simulink model "longtitudinalmodel"  (R2022b)
settings: Solver=VariableStepAuto  StartTime=0.0  StopTime=10.0  FixedStep=0.01  RelTol=1e-3
InitFcn:
  | vehicle_longitudinal_para
values from neighbouring files (symbols this model uses):
  engine_cmd = [0.1, 0.2, 0.3, 0.4, 0.5, 0.4, 0.4, 0.5, 0.4, 0.3]    [vehicle_longitudinal_para.m]
  FR = 1.18    [VehicleLongtitudinalModel.m]    (also in vehicle_longitudinal_para.m)
  generator_cmd = [0, 1, 2, 3, 4, 5, 6, 7, 8, 9] * 5    [vehicle_longitudinal_para.m]
  k = Nr/Ns    (= 2.6)    [VehicleLongtitudinalModel.m]    (also in vehicle_longitudinal_para.m)
  motor_cmd = 1000 + 20 * [0, 1, 2, 3, 4, 5, 6, 7, 8, 9]    [vehicle_longitudinal_para.m]
  R_tire = 0.5    [VehicleLongtitudinalModel.m]    (also in vehicle_longitudinal_para.m)
  testTime = [0, 1, 2, 3, 4, 5, 6, 7, 8, 9]    [vehicle_longitudinal_para.m]
settings Model: Creator=12159  LastModifiedBy=12159

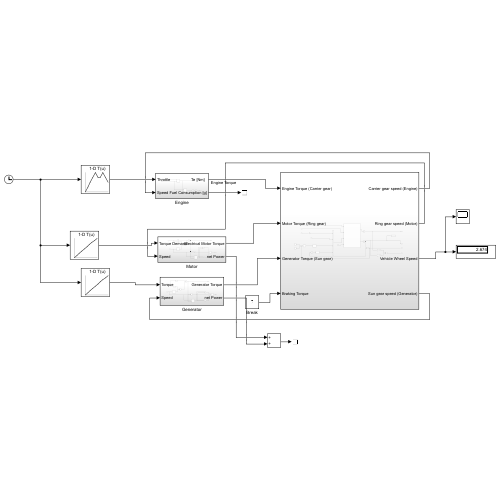
[thumbnail: Simulink's stored preview of the top-level diagram]
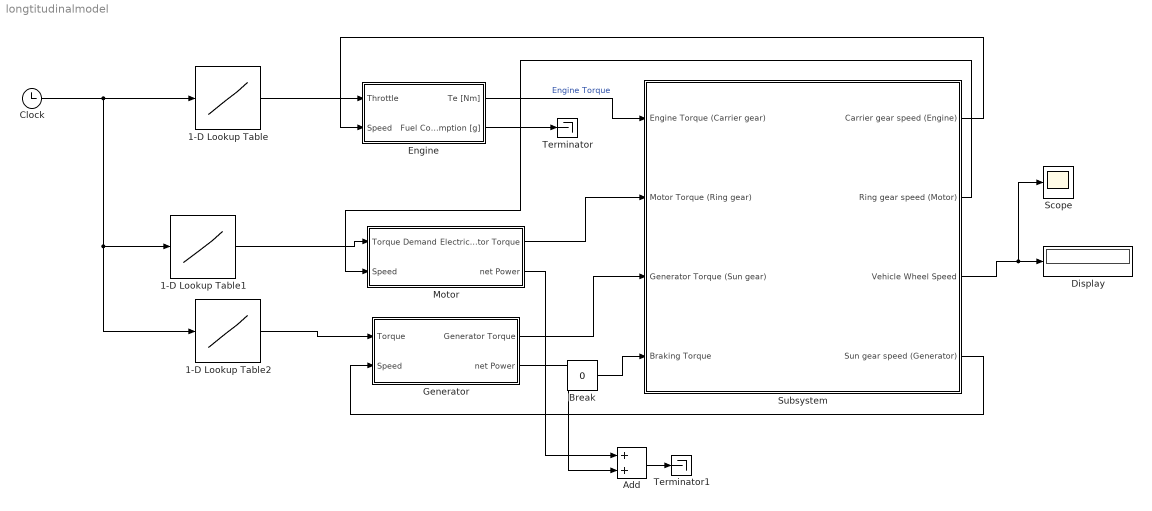
== system longtitudinalmodel ==
  1-D Lookup Table : Lookup_n-D  NumberOfTableDimensions=1  BreakpointsForDimension1=testTime  Table=engine_cmd  InternalRulePriority=Speed  RndMeth=Simplest
  1-D Lookup Table1 : Lookup_n-D  NumberOfTableDimensions=1  BreakpointsForDimension1=testTime  Table=motor_cmd  InternalRulePriority=Speed  RndMeth=Simplest
  1-D Lookup Table2 : Lookup_n-D  NumberOfTableDimensions=1  BreakpointsForDimension1=testTime  Table=generator_cmd  InternalRulePriority=Speed  RndMeth=Simplest
  Add : Sum
  Break : Constant  Value=0
  Clock : Clock
  Display : Display
  Engine : Subsystem
  Generator : Subsystem
  Motor : Subsystem
  Scope : Scope
  Subsystem : Subsystem
  Terminator : Terminator
  Terminator1 : Terminator
  wires:
  Clock/1 -> 1-D Lookup Table/1, 1-D Lookup Table1/1, 1-D Lookup Table2/1
  1-D Lookup Table/1 -> Engine/1(Throttle)
  1-D Lookup Table1/1 -> Motor/1(Torque Demand)
  Motor/2(net Power) -> Add/1
  Generator/2(net Power) -> Add/2
  Add/1 -> Terminator1/1
  1-D Lookup Table2/1 -> Generator/1(Torque)
  Engine/2(Fuel Consumption [g]) -> Terminator/1
  Engine/1("Te [Nm] ") -> Subsystem/1(Engine Torque (Carrier gear))  "Engine Torque"
  Subsystem/1(Carrier gear speed (Engine)) -> Engine/2(Speed)
  Motor/1(Electrical Motor Torque) -> Subsystem/2(Motor Torque (Ring gear))
  Generator/1(Generator Torque) -> Subsystem/3(Generator Torque (Sun gear))
  Break/1 -> Subsystem/4(Braking Torque)
  Subsystem/4(Sun gear speed (Generator)) -> Generator/2(Speed)
  Subsystem/3(Vehicle Wheel Speed) -> Scope/1, Display/1
  Subsystem/2(Ring gear speed (Motor)) -> Motor/2(Speed)

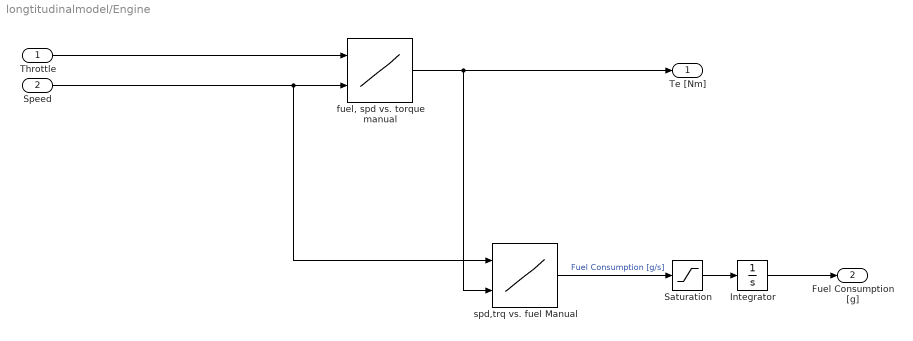
== system longtitudinalmodel/Engine ==
  Throttle : Inport
  Speed : Inport  Port=2
  Integrator : Integrator
  Saturation : Saturate  UpperLimit=1  LowerLimit=0
  "fuel, spd vs. torque manual" : Lookup_n-D  BreakpointsForDimension1=[0 0.1 0.2 0.3 0.4 0.5 0.6 0.7 0.8 0.9 1]  BreakpointsForDimension2=[52.35 55 57.6 60.2 62.85 65.45 68.05 70.7 73.3 75.9 78.55 81.15 83.8 86.4 89 91.65 94.25 96.85 99.5 102.1 104.7 107.35 109.95 112.55 115.2 117.8 120.45 123.05 125.65 128.3 130.9 133.5 136.15 138.75 141.35 144 146.6 149.25 151.85 154.45 157.1 159.7 162.3 164.95 167.55 170.15 172.8 175.4 178 180.65 183.25 185.9 188.5 191.1 193.75 196.35 198.95 201.6 204.2 206.8 209.45]  Table=[0 0 0 0 0 0 0 0 0 0 0 0 0 0 0 0 0 0 0 0 0 0 0 0 0 0 0 0 0 0 0 0 0 0 0 0 0 0 0 0 0 0 0 0 0 0 0 0 0 0 0 0 0 0 0 0 0 0 0 0 0;106.452310717797 107.649950835792 108.847590953786 110.04523107178 111.242871189774 112.440511307768 113.362831858407 114.051130776794 114.739429695182 115.427728613569 116.116027531957 116.776794493609 117.286135693215 117.80924287119 118.318584070796 118.827925270403 119.351032448378 119.942969518191 120.589970501475 121.250737463127 121.897738446411 122.544739429695 123.164208456244 123.604719764012 124.04523107178 124.485742379548 124.940019665683 125.380530973451 125.821042281219 126.275319567355 126.715830875123 127.170108161259 127.610619469027 128.064896755162 128.50540806293 128.945919370698 129.386430678466 129.840707964602 130.28121927237 130.721730580138 131.176007866273 131.616519174041 132.057030481809 132.511307767945 132.951819075713 133.392330383481 133.832841691249 134.287118977384 134.727630285152 135.16814159292 135.622418879056 136.062930186824 136.51720747296 136.957718780728 137.398230088496 137.935103244838 138.34808259587 138.89872173058 139.44936086529 140 140.412979351032;212.904621435595 215.299901671583 217.695181907571 220.09046214356 222.485742379548 224.881022615536 226.725663716814 228.102261553589 229.478859390364 230.855457227139 232.232055063913 233.553588987217 234.572271386431 235.61848574238 236.637168141593 237.655850540806 238.702064896755 239.885939036382 241.17994100295 242.501474926254 243.795476892822 245.08947885939 246.328416912488 247.209439528024 248.09046214356 248.971484759095 249.880039331367 250.761061946903 251.642084562439 252.55063913471 253.431661750246 254.340216322517 255.221238938053 256.129793510324 257.01081612586 257.891838741396 258.772861356932 259.681415929204 260.562438544739 261.443461160275 262.352015732547 263.233038348083 264.114060963618 265.02261553589 265.903638151426 266.784660766962 267.665683382498 268.574237954769 269.455260570305 270.336283185841 271.244837758112 272.125860373648 273.034414945919 273.915437561455 274.796460176991 275.870206489676 276.69616519174 277.79744346116 278.89872173058 280 280.825958702065;319.356932153392 322.949852507375 326.542772861357 330.135693215339 333.728613569322 337.321533923304 340.088495575221 342.153392330383 344.218289085546 346.283185840708 348.34808259587 350.330383480826 351.858407079646 353.427728613569 354.955752212389 356.483775811209 358.053097345133 359.828908554572 361.769911504425 363.75221238938 365.693215339233 367.634218289085 369.492625368732 370.814159292035 372.135693215339 373.457227138643 374.82005899705 376.141592920354 377.463126843658 378.825958702065 380.147492625369 381.510324483776 382.83185840708 384.194690265487 385.516224188791 386.837758112094 388.159292035398 389.522123893805 390.843657817109 392.165191740413 393.52802359882 394.849557522124 396.171091445428 397.533923303835 398.855457227139 400.176991150442 401.498525073746 402.861356932153 404.182890855457 405.504424778761 406.867256637168 408.188790560472 409.551622418879 410.873156342183 412.194690265487 413.805309734513 415.044247787611 416.69616519174 418.34808259587 420 421.238938053097;425.80924287119 430.599803343166 435.390363815143 440.180924287119 444.971484759095 449.762045231072 453.451327433628 456.204523107178 458.957718780728 461.710914454277 464.464110127827 467.107177974435 469.144542772861 471.236971484759 473.274336283186 475.311701081613 477.40412979351 479.771878072763 482.3598820059 485.002949852507 487.590953785644 490.178957718781 492.656833824975 494.418879056047 496.180924287119 497.942969518191 499.760078662734 501.522123893805 503.284169124877 505.10127826942 506.863323500492 508.680432645034 510.442477876106 512.259587020649 514.021632251721 515.783677482793 517.545722713864 519.362831858407 521.124877089479 522.886922320551 524.704031465093 526.466076696165 528.228121927237 530.04523107178 531.807276302852 533.569321533923 535.331366764995 537.148475909538 538.91052114061 ...(+6299 chars)]  InternalRulePriority=Speed  RndMeth=Simplest
      settings: InputPortMap=u0,u1
  spd,trq vs. fuel Manual : Lookup_n-D  BreakpointsForDimension1=[52.35 55 57.6 60.2 62.85 65.45 68.05 70.7 73.3 75.9 78.55 81.15 83.8 86.4 89 91.65 94.25 96.85 99.5 102.1 104.7 107.35 109.95 112.55 115.2 117.8 120.45 123.05 125.65 128.3 130.9 133.5 136.15 138.75 141.35 144 146.6 149.25 151.85 154.45 157.1 159.7 162.3 164.95 167.55 170.15 172.8 175.4 178 180.65 183.25 185.9 188.5 191.1 193.75 196.35 198.95 201.6 204.2 206.8 209.45]  BreakpointsForDimension2=[0 137.659783677483 206.489675516224 275.319567354966 344.149459193707 412.979351032448 481.80924287119 550.639134709931 619.469026548673 688.298918387414 757.128810226155 825.958702064897 894.788593903638 963.618485742379 1032.44837758112 1101.27826941986 1170.1081612586 1238.93805309735 1307.76794493609 1376.59783677483]  Table=[0 3.924 1.968 1.428 1.392 1.542 1.74 1.938 2.118 2.286 2.442 2.61 2.79 3.006 3.27 3.594 3.99 4.476 5.052 5.742;0 4.002 2.052 1.518 1.494 1.65 1.854 2.058 2.25 2.424 2.592 2.76 2.952 3.18 3.45 3.78 4.182 4.674 5.262 5.958;0 4.074 2.13 1.608 1.59 1.752 1.962 2.178 2.376 2.556 2.73 2.91 3.108 3.342 3.618 3.954 4.368 4.866 5.46 6.18;0 4.146 2.208 1.692 1.68 1.848 2.07 2.292 2.496 2.682 2.862 3.054 3.258 3.498 3.78 4.128 4.548 5.052 5.652 6.36;0 4.206 2.28 1.77 1.764 1.944 2.172 2.4 2.61 2.808 2.994 3.186 3.402 3.648 3.942 4.296 4.722 5.232 5.844 6.54;0 4.266 2.346 1.842 1.848 2.052 2.28 2.508 2.706 2.898 3.09 3.324 3.54 3.792 4.092 4.452 4.89 5.406 6 6.72;0 4.326 2.412 1.92 1.926 2.154 2.382 2.616 2.844 3.036 3.228 3.48 3.732 3.936 4.242 4.614 5.052 5.58 6.18 6.96;0 4.386 2.478 1.986 2.004 2.226 2.478 2.718 2.952 3.168 3.354 3.588 3.894 4.08 4.392 4.764 5.214 5.748 6.36 7.14;0 4.44 2.538 2.058 2.082 2.298 2.55 2.796 3.048 3.288 3.474 3.702 4.008 4.302 4.536 4.92 5.37 5.91 6.54 7.32;0 4.494 2.598 2.124 2.154 2.37 2.622 2.868 3.12 3.366 3.582 3.816 4.122 4.428 4.68 5.064 5.526 6.06 6.72 7.5;0 4.548 2.658 2.196 2.232 2.442 2.688 2.94 3.192 3.462 3.666 3.936 4.248 4.56 4.818 5.214 5.682 6.24 6.9 7.62;0 4.602 2.718 2.262 2.304 2.514 2.76 3.012 3.276 3.564 3.768 4.056 4.368 4.686 4.992 5.358 5.832 6.42 7.08 7.8;0 4.656 2.784 2.328 2.376 2.58 2.832 3.096 3.378 3.666 3.888 4.182 4.482 4.8 5.112 5.502 5.982 6.54 7.2 7.98;0 4.71 2.844 2.394 2.454 2.652 2.91 3.198 3.486 3.768 4.014 4.308 4.602 4.914 5.22 5.646 6.12 6.72 7.38 8.16;0 4.77 2.904 2.466 2.526 2.73 3.018 3.3 3.588 3.87 4.14 4.428 4.722 5.028 5.34 5.82 6.3 6.84 7.56 8.34;0 4.824 2.97 2.532 2.544 2.832 3.12 3.402 3.69 3.978 4.272 4.578 4.878 5.184 5.508 5.892 6.42 7.02 7.68 8.46;0 4.884 3.036 2.604 2.676 2.952 3.24 3.528 3.81 4.104 4.428 4.758 5.082 5.406 5.712 6.12 6.6 7.14 7.86 8.64;0 4.944 3.102 2.676 2.778 3.078 3.36 3.648 3.93 4.23 4.554 4.878 5.208 5.532 5.868 6.3 6.84 7.32 8.04 8.82;0 5.004 3.168 2.748 2.808 3.174 3.432 3.768 4.056 4.35 4.68 5.004 5.328 5.67 6 6.42 6.96 7.5 8.16 9;0 5.07 3.24 2.826 2.916 3.192 3.624 3.768 4.176 4.476 4.8 5.13 5.466 5.814 6.18 6.54 7.08 7.62 8.34 9.12;0 5.136 3.312 2.904 3 3.3 3.63 3.954 4.296 4.602 4.926 5.268 5.616 5.964 6.3 6.66 7.2 7.8 8.52 9.3;0 5.208 3.384 2.982 3.084 3.384 3.72 4.05 4.374 4.722 5.07 5.418 5.766 6.12 6.48 6.78 7.32 7.92 8.64 9.48;0 5.28 3.462 3.066 3.174 3.462 3.822 4.134 4.488 4.86 5.214 5.562 5.91 6.24 6.6 6.96 7.5 8.1 8.82 9.66;0 5.352 3.54 3.15 3.264 3.552 3.912 4.248 4.596 5.064 5.34 5.694 6.06 6.42 6.78 7.08 7.62 8.28 9 9.84;0 5.43 3.618 3.234 3.354 3.654 4.002 4.344 4.716 5.304 5.544 5.814 6.18 6.54 6.9 7.26 7.74 8.4 9.12 9.96;0 5.508 3.708 3.324 3.45 3.75 4.104 4.476 4.824 5.562 5.76 6 6.3 6.66 7.02 7.38 7.86 8.58 9.3 10.14;0 5.592 3.792 3.414 3.546 3.852 4.212 4.59 4.95 5.34 5.958 6.24 6.48 6.78 7.14 7.56 8.1 8.7 9.48 10.32;0 5.676 3.882 3.51 3.642 3.96 4.32 4.71 5.058 5.454 6.18 6.48 6.72 6.9 7.26 7.8 8.34 8.82 9.66 10.5;0 5.766 3.978 3.612 3.75 4.068 4.434 4.824 5.166 5.574 6.42 6.66 6.96 7.14 7.44 7.98 8.52 9 9.78 10.68;0 5.856 4.074 3.714 3.852 4.176 4.548 4.92 5.292 5.706 6.66 6.84 7.14 7.38 7.62 8.1 8.64 9.18 9.96 10.86;0 5.952 4.176 3.816 3.96 4.29 4.668 5.046 5.418 5.826 6.264 6.702 7.38 7.62 7.86 8.22 8.76 9.36 10.14 10.98;0 6.06 4.278 3.924 4.074 4.404 4.788 5.166 5.538 5.94 6.39 6.834 7.56 7.86 8.1 8.4 8.88 9.54 10.32 11.16;0 6.18 4.386 4.038 4.188 4.524 4.908 5.298 5.67 6.06 6.516 6.972 7.74 8.04 8.34 8.58 9.06 9.72 10.5 11.34;0 6.24 4.494 4.152 4.308 4.65 5.04 5.43 5.802 6.18 6.642 7.134 7.98 8.28 8.52 8.82 9.18 9.9 10.68 11.52;0 6.36 4.608 4.266 4.428 4.776 5.166 5.562 5.94 6.3 6.762 7.266 8.16 8.46 8.76 9 9.36 10.08 10.86 11.7;0 6.48 4.728 4.392 4.554 4.902 5.298 5.7 6.06 6.42 6.888 7.398 8.4 8.64 8.94 9.24 9.48 10.32 11.04 11.88;0 6.6 4.848 4.518 4.686 5.034 5.436 5.838 6.24 6.6 7.014 7.506 8.004 8.586 9.126 9.42 9.72 10.5 11.22 12.06;0 6.72 4.974 4.644 4.818 5.172 5.58 5.982 6.36 6.72 7.14 ...(+2461 chars)]  InternalRulePriority=Speed  RndMeth=Simplest
      settings: InputPortMap=u0,u1
  "Te [Nm] " : Outport
  Fuel Consumption [g] : Outport  Port=2
  wires:
  Integrator/1 -> Fuel Consumption [g]/1
  "fuel, spd vs. torque manual"/1 -> "Te [Nm] "/1, spd,trq vs. fuel Manual/2
  Throttle/1 -> "fuel, spd vs. torque manual"/1
  Speed/1 -> spd,trq vs. fuel Manual/1, "fuel, spd vs. torque manual"/2
  spd,trq vs. fuel Manual/1 -> Saturation/1  "Fuel Consumption [g/s]"
  Saturation/1 -> Integrator/1

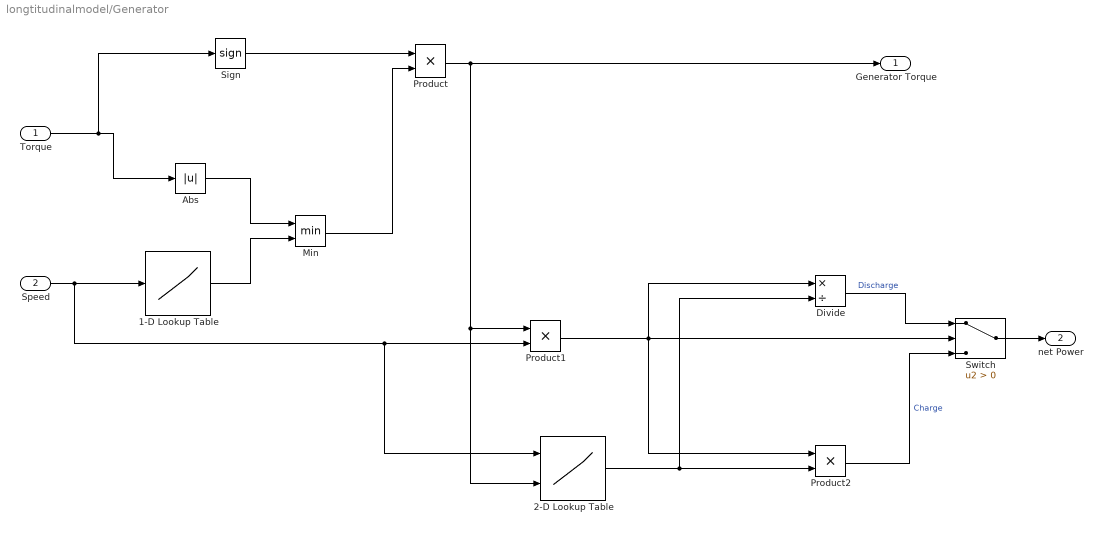
== system longtitudinalmodel/Generator ==
  Torque : Inport
  Speed : Inport  Port=2
  1-D Lookup Table : Lookup_n-D  NumberOfTableDimensions=1  BreakpointsForDimension1=[-20943.951023932 -1047.1975511966 -837.758040957278 -680.678408277789 -575.958653158129 -418.879020478639 -366.519142918809 -314.159265358979 -261.799387799149 -209.43951023932 -157.07963267949 -104.71975511966 -52.3598775598299 0 52.3598775598299 104.71975511966 157.07963267949 209.43951023932 261.799387799149 314.159265358979 366.519142918809 418.879020478639 575.958653158129 680.678408277789 837.758040957278 1047.1975511966 20943.951023932]  Table=[0.012 17.16 21.6 26.4 31.2 43.2 49.2 57.6 66 66 66 66 66 66 66 66 66 66 66 57.6 49.2 43.2 31.2 26.4 21.6 17.16 0.012]  InternalRulePriority=Speed  RndMeth=Simplest
  2-D Lookup Table : Lookup_n-D  BreakpointsForDimension1=[-628.318530717959 -575.958653158129 -418.879020478639 -366.519142918809 -314.159265358979 -261.799387799149 -209.43951023932 -157.07963267949 -104.71975511966 -52.3598775598299 0 52.3598775598299 104.71975511966 157.07963267949 209.43951023932 261.799387799149 314.159265358979 366.519142918809 418.879020478639 575.958653158129 628.318530717959]  BreakpointsForDimension2=[-55 -45 -35 -25 -15 -5 0 5 15 25 35 45 55]  Table=[0.836 0.8455 0.855 0.8645 0.855 0.7505 0.7505 0.7505 0.855 0.8645 0.855 0.8455 0.836;0.836 0.8455 0.855 0.8645 0.855 0.7505 0.7505 0.7505 0.855 0.8645 0.855 0.8455 0.836;0.836 0.8455 0.855 0.8645 0.855 0.7505 0.7505 0.7505 0.855 0.8645 0.855 0.8455 0.836;0.8265 0.836 0.855 0.855 0.855 0.76 0.76 0.76 0.855 0.855 0.855 0.836 0.8265;0.8075 0.8265 0.8455 0.855 0.855 0.7695 0.7695 0.7695 0.855 0.855 0.8455 0.8265 0.8075;0.7885 0.8075 0.8265 0.8455 0.8455 0.779 0.779 0.779 0.8455 0.8455 0.8265 0.8075 0.7885;0.76 0.7885 0.8075 0.8265 0.8455 0.779 0.779 0.779 0.8455 0.8265 0.8075 0.7885 0.76;0.722 0.7505 0.779 0.8075 0.8265 0.779 0.779 0.779 0.8265 0.8075 0.779 0.7505 0.722;0.646 0.684 0.722 0.76 0.798 0.7695 0.76 0.7695 0.798 0.76 0.722 0.684 0.646;0.494 0.5415 0.5985 0.6555 0.7315 0.76 0.76 0.76 0.7315 0.6555 0.5985 0.5415 0.494;0.494 0.5415 0.5985 0.6555 0.7315 0.76 0.76 0.76 0.7315 0.6555 0.5985 0.5415 0.494;0.494 0.5415 0.5985 0.6555 0.7315 0.76 0.76 0.76 0.7315 0.6555 0.5985 0.5415 0.494;0.646 0.684 0.722 0.76 0.798 0.7695 0.76 0.7695 0.798 0.76 0.722 0.684 0.646;0.722 0.7505 0.779 0.8075 0.8265 0.779 0.779 0.779 0.8265 0.8075 0.779 0.7505 0.722;0.76 0.7885 0.8075 0.8265 0.8455 0.779 0.779 0.779 0.8455 0.8265 0.8075 0.7885 0.76;0.7885 0.8075 0.8265 0.8455 0.8455 0.779 0.779 0.779 0.8455 0.8455 0.8265 0.8075 0.7885;0.8075 0.8265 0.8455 0.855 0.855 0.7695 0.7695 0.7695 0.855 0.855 0.8455 0.8265 0.8075;0.8265 0.836 0.855 0.855 0.855 0.76 0.76 0.76 0.855 0.855 0.855 0.836 0.8265;0.836 0.8455 0.855 0.8645 0.855 0.7505 0.7505 0.7505 0.855 0.8645 0.855 0.8455 0.836;0.836 0.8455 0.855 0.8645 0.855 0.7505 0.7505 0.7505 0.855 0.8645 0.855 0.8455 0.836;0.836 0.8455 0.855 0.8645 0.855 0.7505 0.7505 0.7505 0.855 0.8645 0.855 0.8455 0.836]  InternalRulePriority=Speed  RndMeth=Simplest
      settings: InputPortMap=u0,u1
  Abs : Abs  SaturateOnIntegerOverflow=off
  Divide : Product  Inputs=*/
  Min : MinMax  Inputs=2
  Product : Product
  Product1 : Product
  Product2 : Product
  Sign : Signum
  Switch : Switch  Criteria=u2 > Threshold  SaturateOnIntegerOverflow=off  InputSameDT=off
  Generator Torque : Outport
  net Power : Outport  Port=2
  wires:
  Speed/1 -> 2-D Lookup Table/1, Product1/2, 1-D Lookup Table/1
  1-D Lookup Table/1 -> Min/2
  Torque/1 -> Sign/1, Abs/1
  Sign/1 -> Product/1
  Min/1 -> Product/2
  Abs/1 -> Min/1
  Product/1 -> 2-D Lookup Table/2, Product1/1, Generator Torque/1
  2-D Lookup Table/1 -> Divide/2, Product2/2
  Product1/1 -> Product2/1, Divide/1, Switch/2
  Product2/1 -> Switch/3  "Charge"
  Divide/1 -> Switch/1  "Discharge"
  Switch/1 -> net Power/1

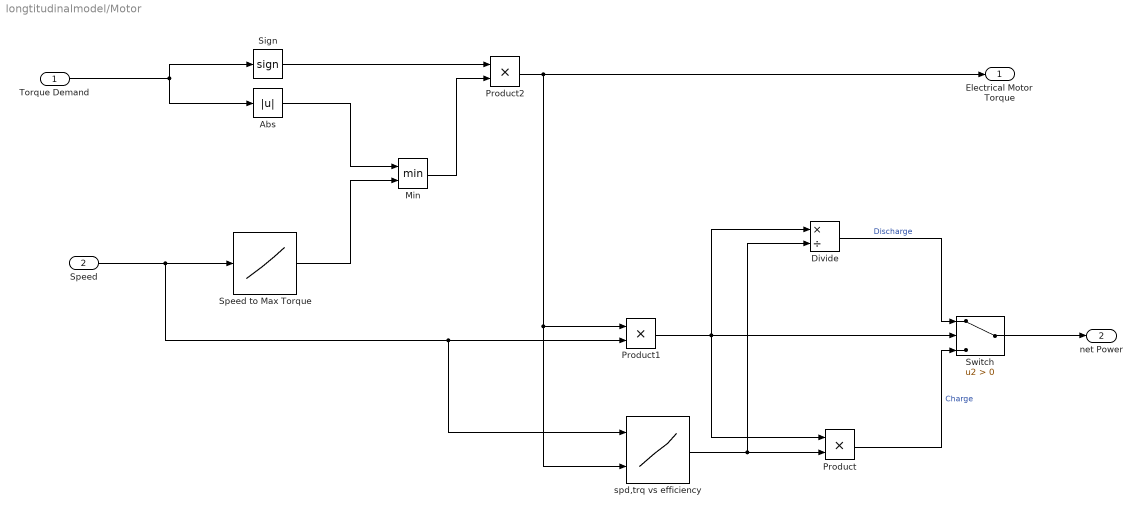
== system longtitudinalmodel/Motor ==
  Torque Demand : Inport
  Speed : Inport  Port=2
  Abs : Abs  SaturateOnIntegerOverflow=off
  Divide : Product  Inputs=*/
  Min : MinMax  Inputs=2
  Product : Product
  Product1 : Product
  Product2 : Product
  Sign : Signum
  Speed to Max Torque : Lookup_n-D  NumberOfTableDimensions=1  BreakpointsForDimension1=[0 52.3598775598299 104.71975511966 157.07963267949 209.43951023932 261.799387799149 314.159265358979 366.519142918809 418.879020478639 471.238898038469 628.318530717959]  Table=[2033.33333333333 2033.33333333333 1929.50354609929 1281.29078014184 959.13475177305 766.099290780142 637.659574468085 546.113475177305 478.099290780142 431.559322033898 318]  InternalRulePriority=Speed  RndMeth=Simplest
  Switch : Switch  Criteria=u2 > Threshold  SaturateOnIntegerOverflow=off  InputSameDT=off
  spd,trq vs efficiency : Lookup_n-D  BreakpointsForDimension1=[0 52.3598775598299 104.71975511966 157.07963267949 209.43951023932 261.799387799149 314.159265358979 366.519142918809 418.879020478639 471.238898038469 628.318530717959]  BreakpointsForDimension2=[-2033.33333333333 -1833.33333333333 -1633.33333333333 -1433.33333333333 -1233.33333333333 -1033.33333333333 -833.333333333333 -633.333333333333 -433.333333333333 -233.333333333333 -33.3333333333333 0 33.3333333333333 233.333333333333 433.333333333333 633.333333333333 833.333333333333 1033.33333333333 1233.33333333333 1433.33333333333 1633.33333333333 1833.33333333333 2033.33333333333]  Table=[0.85975 0.85975 0.85975 0.85975 0.85975 0.85975 0.85975 0.85975 0.85975 0.85975 0.85975 0.85975 0.85975 0.85975 0.85975 0.85975 0.85975 0.85975 0.85975 0.85975 0.85975 0.85975 0.85975;0.532 0.5605 0.589 0.6175 0.646 0.684 0.722 0.76 0.8075 0.855 0.8265 0.85975 0.8265 0.855 0.8075 0.76 0.722 0.684 0.646 0.6175 0.589 0.5605 0.532;0.684 0.703 0.722 0.741 0.7695 0.7885 0.817 0.8455 0.8645 0.893 0.8075 0.85975 0.8075 0.893 0.8645 0.8455 0.817 0.7885 0.7695 0.741 0.722 0.703 0.684;0.684 0.703 0.722 0.741 0.817 0.836 0.855 0.874 0.8835 0.893 0.7885 0.85975 0.7885 0.893 0.8835 0.874 0.855 0.836 0.817 0.741 0.722 0.703 0.684;0.684 0.703 0.722 0.741 0.817 0.836 0.874 0.8835 0.9025 0.9025 0.779 0.85975 0.779 0.9025 0.9025 0.8835 0.874 0.836 0.817 0.741 0.722 0.703 0.684;0.684 0.703 0.722 0.741 0.817 0.836 0.874 0.893 0.9025 0.9025 0.7695 0.85975 0.7695 0.9025 0.9025 0.893 0.874 0.836 0.817 0.741 0.722 0.703 0.684;0.684 0.703 0.722 0.741 0.817 0.836 0.874 0.9025 0.912 0.9025 0.7695 0.85975 0.7695 0.9025 0.912 0.9025 0.874 0.836 0.817 0.741 0.722 0.703 0.684;0.684 0.703 0.722 0.741 0.817 0.836 0.874 0.9025 0.912 0.9025 0.76 0.85975 0.76 0.9025 0.912 0.9025 0.874 0.836 0.817 0.741 0.722 0.703 0.684;0.684 0.703 0.722 0.741 0.817 0.836 0.874 0.9025 0.9025 0.9025 0.76 0.85975 0.76 0.9025 0.9025 0.9025 0.874 0.836 0.817 0.741 0.722 0.703 0.684;0.684 0.703 0.722 0.741 0.817 0.836 0.874 0.9025 0.9025 0.9025 0.7505 0.85975 0.7505 0.9025 0.9025 0.9025 0.874 0.836 0.817 0.741 0.722 0.703 0.684;0.684 0.703 0.722 0.741 0.817 0.836 0.874 0.9025 0.9025 0.9025 0.7505 0.85975 0.7505 0.9025 0.9025 0.9025 0.874 0.836 0.817 0.741 0.722 0.703 0.684]  InternalRulePriority=Speed  RndMeth=Simplest
      settings: InputPortMap=u0,u1
  Electrical Motor Torque : Outport
  net Power : Outport  Port=2
  wires:
  Speed to Max Torque/1 -> Min/2
  Abs/1 -> Min/1
  Torque Demand/1 -> Sign/1, Abs/1
  Sign/1 -> Product2/1
  Min/1 -> Product2/2
  Product2/1 -> Product1/1, spd,trq vs efficiency/2, Electrical Motor Torque/1
  spd,trq vs efficiency/1 -> Divide/2, Product/2
  Switch/1 -> net Power/1
  Speed/1 -> spd,trq vs efficiency/1, Product1/2, Speed to Max Torque/1
  Product1/1 -> Divide/1, Product/1, Switch/2
  Divide/1 -> Switch/1  "Discharge"
  Product/1 -> Switch/3  "Charge"

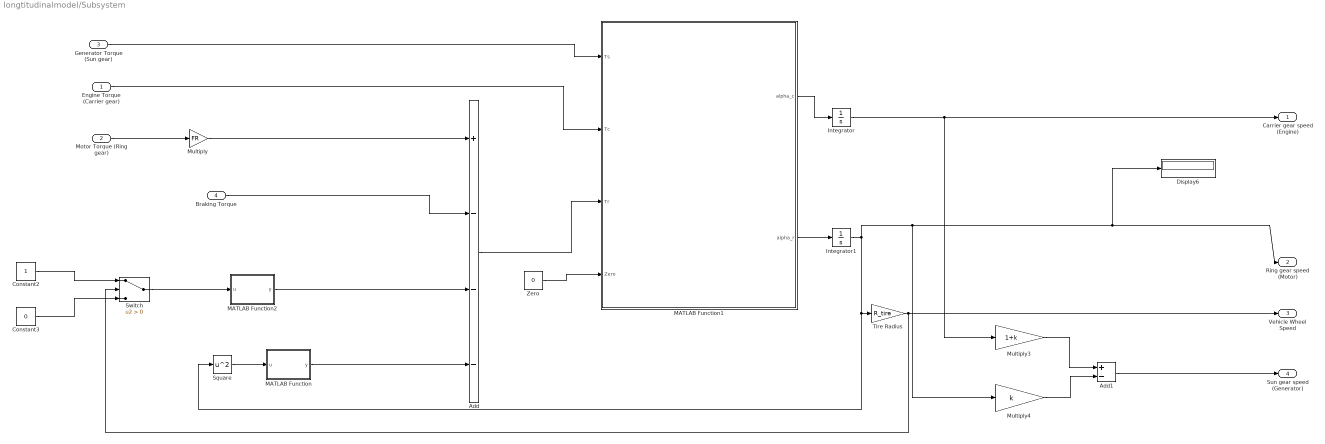
== system longtitudinalmodel/Subsystem ==
  Engine Torque (Carrier gear) : Inport
  Motor Torque (Ring gear) : Inport  Port=2
  Generator Torque (Sun gear) : Inport  Port=3
  Braking Torque : Inport  Port=4
  Add : Sum  Inputs=+---
  Add1 : Sum  Inputs=+-
  Constant2 : Constant
  Constant3 : Constant  Value=0
  Display6 : Display
  Integrator : Integrator
  Integrator1 : Integrator
  MATLAB Function : MATLAB Function  TreatAsAtomicUnit=on
  MATLAB Function1 : MATLAB Function  TreatAsAtomicUnit=on
  MATLAB Function2 : MATLAB Function  TreatAsAtomicUnit=on
  Multiply : Gain  Gain=FR
  Multiply3 : Gain  Gain=1+k
  Multiply4 : Gain  Gain=k
  Square : Math  Operator=square
  Switch : Switch  Criteria=u2 > Threshold  SaturateOnIntegerOverflow=off  InputSameDT=off
  Tire Radius : Gain  Gain=R_tire
  Zero : Constant  Value=0  OutDataTypeStr=Inherit: Inherit via back propagation
  Carrier gear speed (Engine) : Outport
  Ring gear speed (Motor) : Outport  Port=2
  Vehicle Wheel Speed : Outport  Port=3
  Sun gear speed (Generator) : Outport  Port=4
  wires:
  Add1/1 -> Sun gear speed (Generator)/1
  Generator Torque (Sun gear)/1 -> MATLAB Function1/1(Ts)
  MATLAB Function1/2(alpha_r) -> Integrator1/1
  Multiply4/1 -> Add1/2
  MATLAB Function1/1(alpha_c) -> Integrator/1
  Integrator1/1 -> Multiply4/1, Display6/1, Ring gear speed (Motor)/1, Square/1, Tire Radius/1
  MATLAB Function2/1(y) -> Add/3
  Engine Torque (Carrier gear)/1 -> MATLAB Function1/2(Tc)
  Tire Radius/1 -> Switch/2, Vehicle Wheel Speed/1
  Multiply3/1 -> Add1/1
  Motor Torque (Ring gear)/1 -> Multiply/1
  Integrator/1 -> Multiply3/1, Carrier gear speed (Engine)/1
  Zero/1 -> MATLAB Function1/4(Zero)
  Constant2/1 -> Switch/1
  Braking Torque/1 -> Add/2
  Multiply/1 -> Add/1
  Add/1 -> MATLAB Function1/3(Tr)
  Constant3/1 -> Switch/3
  Square/1 -> MATLAB Function/1(u)
  MATLAB Function/1(y) -> Add/4
  Switch/1 -> MATLAB Function2/1(u)

== matlab function longtitudinalmodel/Subsystem/MATLAB Function1 ==
  data: Ts input; alpha_c output; Tc input; Tr input; Zero input; alpha_r output; VehiclePara parameter
function [alpha_c, alpha_r] = Torque2AngularAcc(Ts, Tc, Tr, Zero, VehiclePara)

Is = VehiclePara.Is;
Ig = VehiclePara.Ig;
Ic = VehiclePara.Ic;
Ie = VehiclePara.Ie;
Vehicle_mass = VehiclePara.mass;
R_tire = VehiclePara.R_tire;
FR = VehiclePara.FR;
Im = VehiclePara.Im;
Ir = VehiclePara.Ir;
Ns = VehiclePara.Ns;
Nr = VehiclePara.Nr;
N = VehiclePara.N;

W2T= [Is+Ig     0       0                                        -Ns*N;
        0       Ic+Ie   0                                    (Ns+Nr)*N;
        0       0       Vehicle_mass*R_tire^2/FR+Im*FR+Ir*FR  -FR*Nr*N;
        Ns      -(Ns+Nr) Nr                                         0];
Output = W2T* [Ts; Tc; Tr; Zero];
alpha_c = Output(2);
alpha_r = Output(3);

== matlab function longtitudinalmodel/Subsystem/MATLAB Function ==
  data: u input; y output
function y = fcn(u)
Vehicle_mass = 15076; % vehicle total mass, kg
g = 9.81; % Gravity constant
Cr = 0.0085; % Rolling resistance constant
R_tire = 0.5; % Radius of the tire, m

A_front = 9.5; % Area of the front, m^2
Cd = 0.7963; % Aero drag coefficient
rho_air = 1.2; % Air density kg/m^3

FR = 1.18; % final drive gear ratio
y = 0.5*A_front*rho_air*Cd*R_tire^2/FR*u^2;

== matlab function longtitudinalmodel/Subsystem/MATLAB Function2 ==
  data: u input; y output
function y = fcn(u)
Vehicle_mass = 15076; % vehicle total mass, kg
g = 9.81; % Gravity constant
Cr = 0.0085; % Rolling resistance constant
R_tire = 0.5; % Radius of the tire, m

A_front = 9.5; % Area of the front, m^2
Cd = 0.7963; % Aero drag coefficient
rho_air = 1.2; % Air density kg/m^3

FR = 1.18; % final drive gear ratio
y = Vehicle_mass*g*Cr*R_tire+u;
